simulink model "VisionHelicopter"  (R2025b)
settings: Solver=VariableStepAuto  StartTime=0.0  StopTime=65  RelTol=1e-3
libraries: slpidlib x3
settings Model: Creator=g3sha  LastModifiedBy=g3sha

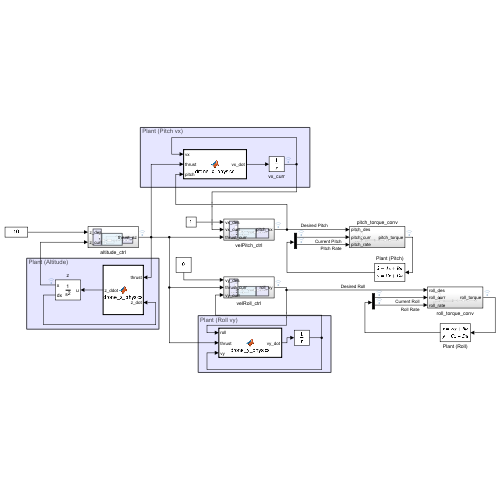
[thumbnail: Simulink's stored preview of the top-level diagram]
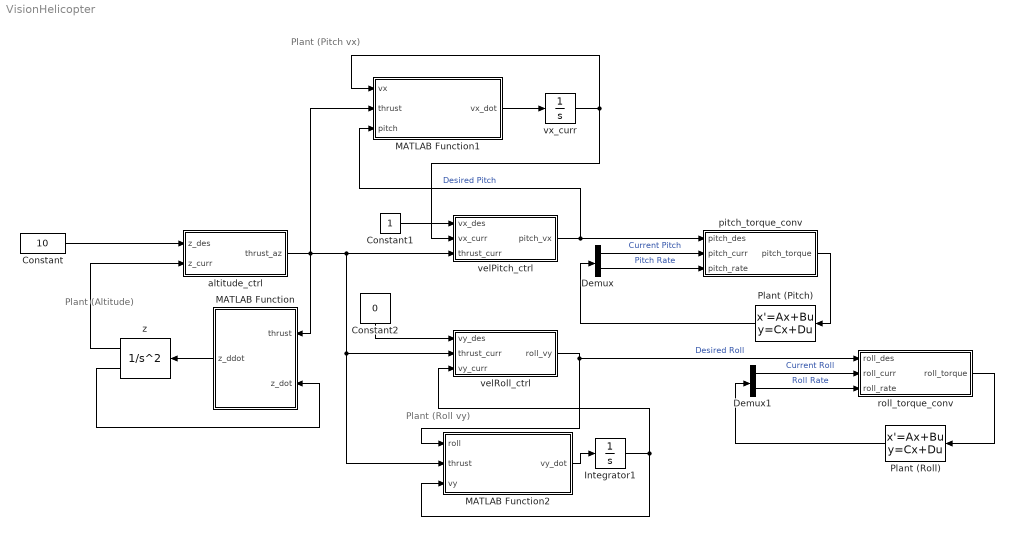
== system VisionHelicopter ==
  note: Plant (Roll vy)
  note: Plant (Pitch vx)
  note: Plant (Altitude)
  Constant : Constant  Value=10
  Constant1 : Constant
  Constant2 : Constant  Value=0
  Demux : Demux  Outputs=2
  Demux1 : Demux  Outputs=2
  Integrator1 : Integrator
  MATLAB Function : MATLAB Function  TreatAsAtomicUnit=on
  MATLAB Function1 : MATLAB Function  TreatAsAtomicUnit=on
  MATLAB Function2 : MATLAB Function  TreatAsAtomicUnit=on
  Plant (Pitch) : StateSpace  A=[0 1; 0 -0.01/0.03125];  B=[0; 1/0.03125];  C=eye(2);  D=[0; 0];  InitialCondition=0
  Plant (Roll) : StateSpace  A=[0 1; 0 -0.01/0.03125];  B=[0; 1/0.03125];  C=eye(2);  D=[0; 0];  InitialCondition=0
  altitude_ctrl : Subsystem
  pitch_torque_conv : Subsystem
  roll_torque_conv : Subsystem
  velPitch_ctrl : Subsystem
  velRoll_ctrl : Subsystem
  vx_curr : Integrator
  z : SecondOrderIntegrator
  wires:
  z/2 -> MATLAB Function/2(z_dot)
  MATLAB Function/1(z_ddot) -> z/1
  z/1 -> altitude_ctrl/2(z_curr)
  altitude_ctrl/1(thrust_az) -> MATLAB Function1/2(thrust), MATLAB Function2/2(thrust), velRoll_ctrl/2(thrust_curr), velPitch_ctrl/3(thrust_curr), MATLAB Function/1(thrust)
  MATLAB Function1/1(vx_dot) -> vx_curr/1
  velPitch_ctrl/1(pitch_vx) -> pitch_torque_conv/1(pitch_des), MATLAB Function1/3(pitch)  "Desired Pitch"
  vx_curr/1 -> velPitch_ctrl/2(vx_curr), MATLAB Function1/1(vx)
  velRoll_ctrl/1(roll_vy) -> roll_torque_conv/1(roll_des), MATLAB Function2/1(roll)  "Desired Roll"
  MATLAB Function2/1(vy_dot) -> Integrator1/1
  Integrator1/1 -> MATLAB Function2/3(vy), velRoll_ctrl/3(vy_curr)
  pitch_torque_conv/1(pitch_torque) -> Plant (Pitch)/1
  Plant (Pitch)/1 -> Demux/1
  Demux/1 -> pitch_torque_conv/2(pitch_curr)  "Current Pitch"
  Demux/2 -> pitch_torque_conv/3(pitch_rate)  "Pitch Rate"
  Constant1/1 -> velPitch_ctrl/1(vx_des)
  Demux1/2 -> roll_torque_conv/3(roll_rate)  "Roll Rate"
  Plant (Roll)/1 -> Demux1/1
  roll_torque_conv/1(roll_torque) -> Plant (Roll)/1
  Demux1/1 -> roll_torque_conv/2(roll_curr)  "Current Roll"
  Constant2/1 -> velRoll_ctrl/1(vy_des)
  Constant/1 -> altitude_ctrl/1(z_des)

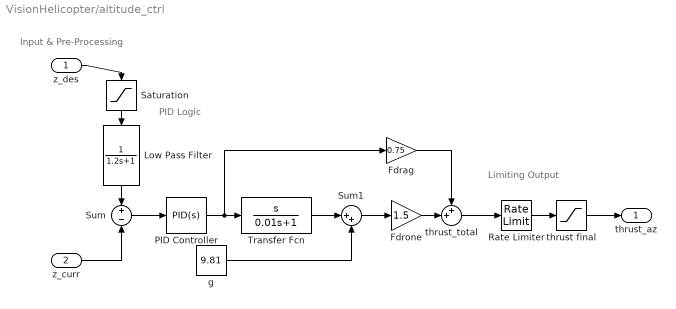
== system VisionHelicopter/altitude_ctrl ==
  note: Limiting Output
  note: PID Logic
  note: Input & Pre-Processing
  z_des : Inport
  z_curr : Inport  Port=2
  Fdrag : Gain  Gain=0.75
  Fdrone : Gain  Gain=1.5
  Low Pass Filter : TransferFcn  Denominator=[1.2 1]
  PID Controller : slpidlib/PID Controller  Controller=PID  Form=Parallel  TimeDomain=Continuous-time  UseExternalTs=off  SampleTime=-1  IntegratorMethod=Forward Euler  FilterMethod=Forward Euler  ControllerParametersSource=internal  P=3  I=2  UseKiTs=off  D=0  UseExternalDerivativeSource=off  N=100  UseFilter=on  TunerSelectOption=Transfer Function Based (PID Tuner App)  InitialConditionSource=internal  InitialConditionForIntegrator=0  InitialConditionForFilter=0  DifferentiatorICPrevScaledInput=0  ExternalReset=none  TrackingMode=off  Kt=1  LimitOutput=off  SatLimitsSource=internal  UpperSaturationLimit=inf  LowerSaturationLimit=-inf  LinearizeAsGain=on  AntiWindupMode=none  Kb=1  LimitIntegrator=on  UpperIntegratorSaturationLimit=5.0  LowerIntegratorSaturationLimit=-5.0  POutMin=[]  POutMax=[]  IOutMin=[]  IOutMax=[]  DOutMin=[]  DOutMax=[]  NOutMin=[]  NOutMax=[]  SumOutMin=[]  SumOutMax=[]  SaturationOutMin=[]  SaturationOutMax=[]  PParamMin=[]  PParamMax=[]  IParamMin=[]  IParamMax=[]  DParamMin=[]  DParamMax=[]  NParamMin=[]  NParamMax=[]  KbParamMin=[]  KbParamMax=[]  KtParamMin=[]  KtParamMax=[]  KbOutMin=[]  KbOutMax=[]  KtOutMin=[]  KtOutMax=[]  IntegratorOutMin=[]  IntegratorOutMax=[]  FilterOutMin=[]  FilterOutMax=[]  SumI1OutMin=[]  SumI1OutMax=[]  SumI2OutMin=[]  SumI2OutMax=[]  SumI3OutMin=[]  SumI3OutMax=[]  SumI4OutMin=[]  SumI4OutMax=[]  SumDOutMin=[]  SumDOutMax=[]  DifferentiatorOutMin=[]  DifferentiatorOutMax=[]  FilterDiffOutCoefMin=[]  FilterDiffOutCoefMax=[]  ReciprocalOutMin=[]  ReciprocalOutMax=[]  SumDenOutMin=[]  SumDenOutMax=[]  SumNumOutMin=[]  SumNumOutMax=[]  DivideOutMin=[]  DivideOutMax=[]  UdiffTsProdOutMin=[]  UdiffTsProdOutMax=[]  NTsProdOutMin=[]  NTsProdOutMax=[]  UintegralTsProdOutMin=[]  UintegralTsProdOutMax=[]  UngainTsProdOutMin=[]  UngainTsProdOutMax=[]  ClampingZeroOutDataTypeStr=Inherit: Inherit via back propagation  ClampingZeroOutMin=[]  ClampingZeroOutMax=[]  FilterDenConstantOutDataTypeStr=Inherit: Inherit via back propagation  FilterDenConstantOutMin=[]  FilterDenConstantOutMax=[]  PCopyOutDataTypeStr=Inherit: Inherit via back propagation  PCopyOutMin=[]  PCopyOutMax=[]  NCopyOutDataTypeStr=Inherit: Inherit via back propagation  NCopyOutMin=[]  NCopyOutMax=[]  IntegratorContinuousStateAttributes=''  IntegratorStateMustResolveToSignalObject=off  IntegratorRTWStateStorageClass=Auto  FilterContinuousStateAttributes=''  FilterStateMustResolveToSignalObject=off  FilterRTWStateStorageClass=Auto  ParallelPVariant=InternalParameters  IdealPVariant=Disabled  IVariant=InternalParameters  DVariant=InternalParameters  IntegratorVariant=Continuous  SatVariant=Disabled  AWVariant=Passthrough  PCopyVariant=Disabled  TRVariant=Disabled  FdbkBlocksVariant=Forward  IdealPFdbkVariant=Disabled  SatFdbkVariant=Disabled  DerivativeFilterVariant=ContFilter  NVariant=InternalParameters  NCopyVariant=Disabled  FilterICVariant=InternalICsFilter  IntegratorICVariant=InternalICs  ExternalResetVariant=Disabled  TRSumVariant=Passthrough  SumFdbkVariant=Disabled  SumVariant=Sum_PID  TsampFilterVariant=InternalTs  TsampNgainVariant=Passthrough  TsampIntegralVariant=Disabled_SignalSpec  ExternalSaturationOutDataTypeStr=Inherit: Same as second input  DerivativeSourceVariant=ErrorSignal  PreIntVariant=InternalPreInt
  Rate Limiter : RateLimiter  RisingSlewLimit=60  FallingSlewLimit=-60  SampleTimeMode=inherited
  Saturation : Saturate  UpperLimit=inf  LowerLimit=0.2
  Sum : Sum  Inputs=+|-
  Sum1 : Sum  Inputs=|++
  Transfer Fcn : TransferFcn  Numerator=[1 0]  Denominator=[0.01 1]
  g : Constant  Value=9.81
  thrust final : Saturate  UpperLimit=20  LowerLimit=2  ZeroCross=off
  thrust_total : Sum  Inputs=++|
  thrust_az : Outport
  wires:
  Sum/1 -> PID Controller/1
  PID Controller/1 -> Transfer Fcn/1, Fdrag/1
  g/1 -> Sum1/2
  Sum1/1 -> Fdrone/1
  Fdrone/1 -> thrust_total/2
  Fdrag/1 -> thrust_total/1
  thrust final/1 -> thrust_az/1
  Transfer Fcn/1 -> Sum1/1
  Rate Limiter/1 -> thrust final/1
  thrust_total/1 -> Rate Limiter/1
  z_curr/1 -> Sum/2
  Saturation/1 -> Low Pass Filter/1
  Low Pass Filter/1 -> Sum/1
  z_des/1 -> Saturation/1

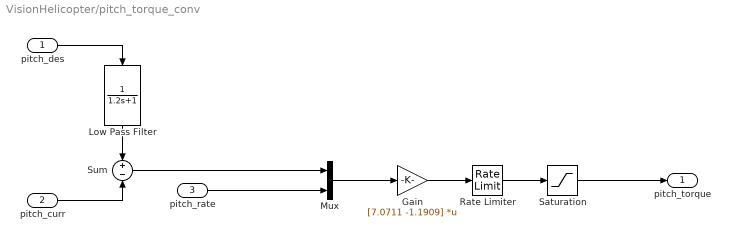
== system VisionHelicopter/pitch_torque_conv ==
  pitch_des : Inport
  pitch_curr : Inport  Port=2
  pitch_rate : Inport  Port=3
  Gain : Gain  Gain=[7.0711 -1.1909]  Multiplication=Matrix(K*u)
  Low Pass Filter : TransferFcn  Denominator=[1.2 1]
  Mux : Mux  Inputs=2
  Rate Limiter : RateLimiter  RisingSlewLimit=3  FallingSlewLimit=-3  SampleTimeMode=inherited
  Saturation : Saturate  UpperLimit=1.5  LowerLimit=-1.5
  Sum : Sum  Inputs=+|-
  pitch_torque : Outport
  wires:
  pitch_curr/1 -> Sum/2
  Sum/1 -> Mux/1
  pitch_rate/1 -> Mux/2
  Mux/1 -> Gain/1
  Gain/1 -> Rate Limiter/1
  Rate Limiter/1 -> Saturation/1
  Saturation/1 -> pitch_torque/1
  Low Pass Filter/1 -> Sum/1
  pitch_des/1 -> Low Pass Filter/1

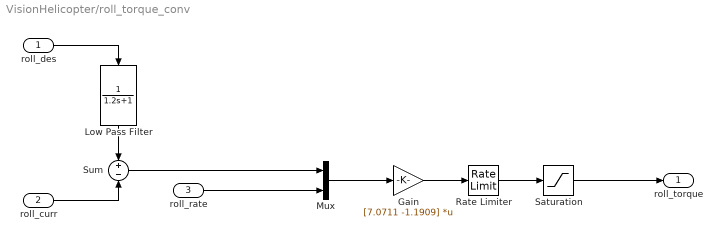
== system VisionHelicopter/roll_torque_conv ==
  roll_des : Inport
  roll_curr : Inport  Port=2
  roll_rate : Inport  Port=3
  Gain : Gain  Gain=[7.0711 -1.1909]  Multiplication=Matrix(K*u)
  Low Pass Filter : TransferFcn  Denominator=[1.2 1]
  Mux : Mux  Inputs=2
  Rate Limiter : RateLimiter  RisingSlewLimit=3  FallingSlewLimit=-3  SampleTimeMode=inherited
  Saturation : Saturate  UpperLimit=1.5  LowerLimit=-1.5
  Sum : Sum  Inputs=+|-
  roll_torque : Outport
  wires:
  roll_curr/1 -> Sum/2
  Sum/1 -> Mux/1
  roll_rate/1 -> Mux/2
  Mux/1 -> Gain/1
  Gain/1 -> Rate Limiter/1
  Rate Limiter/1 -> Saturation/1
  Saturation/1 -> roll_torque/1
  Low Pass Filter/1 -> Sum/1
  roll_des/1 -> Low Pass Filter/1

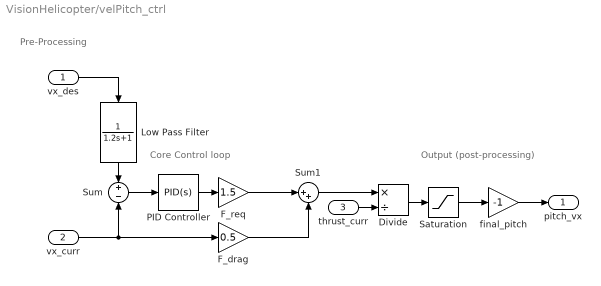
== system VisionHelicopter/velPitch_ctrl ==
  note: Output (post-processing)
  note: Core Control loop
  note: Pre-Processing
  vx_des : Inport
  vx_curr : Inport  Port=2
  thrust_curr : Inport  Port=3
  Divide : Product  Inputs=*/
  F_drag : Gain  Gain=0.5
  F_req : Gain  Gain=1.5
  Low Pass Filter : TransferFcn  Denominator=[1.2 1]
  PID Controller : slpidlib/PID Controller  Controller=PID  Form=Parallel  TimeDomain=Continuous-time  UseExternalTs=off  SampleTime=-1  IntegratorMethod=Forward Euler  FilterMethod=Forward Euler  ControllerParametersSource=internal  P=1  I=1  UseKiTs=off  D=0  UseExternalDerivativeSource=off  N=100  UseFilter=on  TunerSelectOption=Transfer Function Based (PID Tuner App)  InitialConditionSource=internal  InitialConditionForIntegrator=0  InitialConditionForFilter=0  DifferentiatorICPrevScaledInput=0  ExternalReset=none  TrackingMode=off  Kt=1  LimitOutput=off  SatLimitsSource=internal  UpperSaturationLimit=inf  LowerSaturationLimit=-inf  LinearizeAsGain=on  AntiWindupMode=none  Kb=1  LimitIntegrator=on  UpperIntegratorSaturationLimit=5.0  LowerIntegratorSaturationLimit=-5.0  POutMin=[]  POutMax=[]  IOutMin=[]  IOutMax=[]  DOutMin=[]  DOutMax=[]  NOutMin=[]  NOutMax=[]  SumOutMin=[]  SumOutMax=[]  SaturationOutMin=[]  SaturationOutMax=[]  PParamMin=[]  PParamMax=[]  IParamMin=[]  IParamMax=[]  DParamMin=[]  DParamMax=[]  NParamMin=[]  NParamMax=[]  KbParamMin=[]  KbParamMax=[]  KtParamMin=[]  KtParamMax=[]  KbOutMin=[]  KbOutMax=[]  KtOutMin=[]  KtOutMax=[]  IntegratorOutMin=[]  IntegratorOutMax=[]  FilterOutMin=[]  FilterOutMax=[]  SumI1OutMin=[]  SumI1OutMax=[]  SumI2OutMin=[]  SumI2OutMax=[]  SumI3OutMin=[]  SumI3OutMax=[]  SumI4OutMin=[]  SumI4OutMax=[]  SumDOutMin=[]  SumDOutMax=[]  DifferentiatorOutMin=[]  DifferentiatorOutMax=[]  FilterDiffOutCoefMin=[]  FilterDiffOutCoefMax=[]  ReciprocalOutMin=[]  ReciprocalOutMax=[]  SumDenOutMin=[]  SumDenOutMax=[]  SumNumOutMin=[]  SumNumOutMax=[]  DivideOutMin=[]  DivideOutMax=[]  UdiffTsProdOutMin=[]  UdiffTsProdOutMax=[]  NTsProdOutMin=[]  NTsProdOutMax=[]  UintegralTsProdOutMin=[]  UintegralTsProdOutMax=[]  UngainTsProdOutMin=[]  UngainTsProdOutMax=[]  ClampingZeroOutDataTypeStr=Inherit: Inherit via back propagation  ClampingZeroOutMin=[]  ClampingZeroOutMax=[]  FilterDenConstantOutDataTypeStr=Inherit: Inherit via back propagation  FilterDenConstantOutMin=[]  FilterDenConstantOutMax=[]  PCopyOutDataTypeStr=Inherit: Inherit via back propagation  PCopyOutMin=[]  PCopyOutMax=[]  NCopyOutDataTypeStr=Inherit: Inherit via back propagation  NCopyOutMin=[]  NCopyOutMax=[]  IntegratorContinuousStateAttributes=''  IntegratorStateMustResolveToSignalObject=off  IntegratorRTWStateStorageClass=Auto  FilterContinuousStateAttributes=''  FilterStateMustResolveToSignalObject=off  FilterRTWStateStorageClass=Auto  ParallelPVariant=InternalParameters  IdealPVariant=Disabled  IVariant=InternalParameters  DVariant=InternalParameters  IntegratorVariant=Continuous  SatVariant=Disabled  AWVariant=Passthrough  PCopyVariant=Disabled  TRVariant=Disabled  FdbkBlocksVariant=Forward  IdealPFdbkVariant=Disabled  SatFdbkVariant=Disabled  DerivativeFilterVariant=ContFilter  NVariant=InternalParameters  NCopyVariant=Disabled  FilterICVariant=InternalICsFilter  IntegratorICVariant=InternalICs  ExternalResetVariant=Disabled  TRSumVariant=Passthrough  SumFdbkVariant=Disabled  SumVariant=Sum_PID  TsampFilterVariant=InternalTs  TsampNgainVariant=Passthrough  TsampIntegralVariant=Disabled_SignalSpec  ExternalSaturationOutDataTypeStr=Inherit: Same as second input  DerivativeSourceVariant=ErrorSignal  PreIntVariant=InternalPreInt
  Saturation : Saturate  UpperLimit=0.87266  LowerLimit=-0.87266
  Sum : Sum  Inputs=+|-
  Sum1 : Sum  Inputs=|++
  final_pitch : Gain  Gain=-1
  pitch_vx : Outport
  wires:
  vx_curr/1 -> F_drag/1, Sum/2
  Sum/1 -> PID Controller/1
  PID Controller/1 -> F_req/1
  F_req/1 -> Sum1/1
  F_drag/1 -> Sum1/2
  Sum1/1 -> Divide/1
  thrust_curr/1 -> Divide/2
  Divide/1 -> Saturation/1
  Saturation/1 -> final_pitch/1
  final_pitch/1 -> pitch_vx/1
  Low Pass Filter/1 -> Sum/1
  vx_des/1 -> Low Pass Filter/1

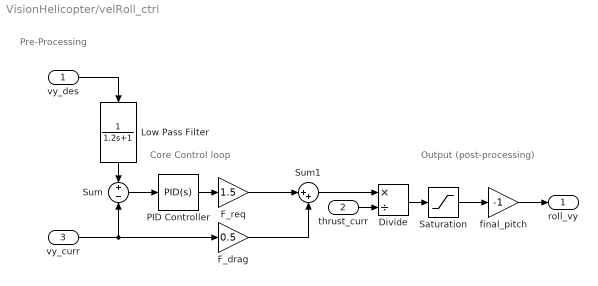
== system VisionHelicopter/velRoll_ctrl ==
  note: Output (post-processing)
  note: Core Control loop
  note: Pre-Processing
  vy_des : Inport
  thrust_curr : Inport  Port=2
  vy_curr : Inport  Port=3
  Divide : Product  Inputs=*/
  F_drag : Gain  Gain=0.5
  F_req : Gain  Gain=1.5
  Low Pass Filter : TransferFcn  Denominator=[1.2 1]
  PID Controller : slpidlib/PID Controller  Controller=PID  Form=Parallel  TimeDomain=Continuous-time  UseExternalTs=off  SampleTime=-1  IntegratorMethod=Forward Euler  FilterMethod=Forward Euler  ControllerParametersSource=internal  P=1  I=1  UseKiTs=off  D=0  UseExternalDerivativeSource=off  N=100  UseFilter=on  TunerSelectOption=Transfer Function Based (PID Tuner App)  InitialConditionSource=internal  InitialConditionForIntegrator=0  InitialConditionForFilter=0  DifferentiatorICPrevScaledInput=0  ExternalReset=none  TrackingMode=off  Kt=1  LimitOutput=off  SatLimitsSource=internal  UpperSaturationLimit=inf  LowerSaturationLimit=-inf  LinearizeAsGain=on  AntiWindupMode=none  Kb=1  LimitIntegrator=on  UpperIntegratorSaturationLimit=5.0  LowerIntegratorSaturationLimit=-5.0  POutMin=[]  POutMax=[]  IOutMin=[]  IOutMax=[]  DOutMin=[]  DOutMax=[]  NOutMin=[]  NOutMax=[]  SumOutMin=[]  SumOutMax=[]  SaturationOutMin=[]  SaturationOutMax=[]  PParamMin=[]  PParamMax=[]  IParamMin=[]  IParamMax=[]  DParamMin=[]  DParamMax=[]  NParamMin=[]  NParamMax=[]  KbParamMin=[]  KbParamMax=[]  KtParamMin=[]  KtParamMax=[]  KbOutMin=[]  KbOutMax=[]  KtOutMin=[]  KtOutMax=[]  IntegratorOutMin=[]  IntegratorOutMax=[]  FilterOutMin=[]  FilterOutMax=[]  SumI1OutMin=[]  SumI1OutMax=[]  SumI2OutMin=[]  SumI2OutMax=[]  SumI3OutMin=[]  SumI3OutMax=[]  SumI4OutMin=[]  SumI4OutMax=[]  SumDOutMin=[]  SumDOutMax=[]  DifferentiatorOutMin=[]  DifferentiatorOutMax=[]  FilterDiffOutCoefMin=[]  FilterDiffOutCoefMax=[]  ReciprocalOutMin=[]  ReciprocalOutMax=[]  SumDenOutMin=[]  SumDenOutMax=[]  SumNumOutMin=[]  SumNumOutMax=[]  DivideOutMin=[]  DivideOutMax=[]  UdiffTsProdOutMin=[]  UdiffTsProdOutMax=[]  NTsProdOutMin=[]  NTsProdOutMax=[]  UintegralTsProdOutMin=[]  UintegralTsProdOutMax=[]  UngainTsProdOutMin=[]  UngainTsProdOutMax=[]  ClampingZeroOutDataTypeStr=Inherit: Inherit via back propagation  ClampingZeroOutMin=[]  ClampingZeroOutMax=[]  FilterDenConstantOutDataTypeStr=Inherit: Inherit via back propagation  FilterDenConstantOutMin=[]  FilterDenConstantOutMax=[]  PCopyOutDataTypeStr=Inherit: Inherit via back propagation  PCopyOutMin=[]  PCopyOutMax=[]  NCopyOutDataTypeStr=Inherit: Inherit via back propagation  NCopyOutMin=[]  NCopyOutMax=[]  IntegratorContinuousStateAttributes=''  IntegratorStateMustResolveToSignalObject=off  IntegratorRTWStateStorageClass=Auto  FilterContinuousStateAttributes=''  FilterStateMustResolveToSignalObject=off  FilterRTWStateStorageClass=Auto  ParallelPVariant=InternalParameters  IdealPVariant=Disabled  IVariant=InternalParameters  DVariant=InternalParameters  IntegratorVariant=Continuous  SatVariant=Disabled  AWVariant=Passthrough  PCopyVariant=Disabled  TRVariant=Disabled  FdbkBlocksVariant=Forward  IdealPFdbkVariant=Disabled  SatFdbkVariant=Disabled  DerivativeFilterVariant=ContFilter  NVariant=InternalParameters  NCopyVariant=Disabled  FilterICVariant=InternalICsFilter  IntegratorICVariant=InternalICs  ExternalResetVariant=Disabled  TRSumVariant=Passthrough  SumFdbkVariant=Disabled  SumVariant=Sum_PID  TsampFilterVariant=InternalTs  TsampNgainVariant=Passthrough  TsampIntegralVariant=Disabled_SignalSpec  ExternalSaturationOutDataTypeStr=Inherit: Same as second input  DerivativeSourceVariant=ErrorSignal  PreIntVariant=InternalPreInt
  Saturation : Saturate  UpperLimit=0.87266  LowerLimit=-0.87266
  Sum : Sum  Inputs=+|-
  Sum1 : Sum  Inputs=|++
  final_pitch : Gain  Gain=-1
  roll_vy : Outport
  wires:
  vy_curr/1 -> F_drag/1, Sum/2
  Sum/1 -> PID Controller/1
  PID Controller/1 -> F_req/1
  F_req/1 -> Sum1/1
  F_drag/1 -> Sum1/2
  Sum1/1 -> Divide/1
  thrust_curr/1 -> Divide/2
  Divide/1 -> Saturation/1
  Saturation/1 -> final_pitch/1
  final_pitch/1 -> roll_vy/1
  Low Pass Filter/1 -> Sum/1
  vy_des/1 -> Low Pass Filter/1

== matlab function VisionHelicopter/MATLAB Function ==
  data: thrust input; z_ddot output; z_dot input
function z_ddot = drone_z_physics(thrust, z_dot)
    m = 1.50;      
    g = 9.81;      
    c = 0.50;      
    
    % second law of motion: a = F_net / m
    F_gravity = m * g;
    F_drag = c * z_dot;
    
    z_ddot = (thrust - F_gravity - F_drag) / m;
end

== matlab function VisionHelicopter/MATLAB Function2 ==
  data: roll input; thrust input; vy input; vy_dot output
function vy_dot = drone_y_physics(roll, thrust, vy)
    % Parameters
    m = 1.50;      
    c = 0.50;      
    
    F_y = -thrust * sin(roll);
    F_drag = c * vy;

    vy_dot = (F_y - F_drag) / m;
end

== matlab function VisionHelicopter/MATLAB Function1 ==
  data: vx input; thrust input; pitch input; vx_dot output
function vx_dot = drone_x_physics(vx, thrust, pitch)
    % Parameters
    m = 1.50;      
    c = 0.50;      
    
    F_x = -thrust * sin(pitch);
    F_drag = c * vx;

    vx_dot = (F_x - F_drag) / m;
end
